simulink model "problem2b_sim_copy"  (R2024b)
settings: Solver=VariableStepAuto  StartTime=0.0  StopTime=2  FixedStep=0.04  RelTol=1e-3  AbsTol=1e-3  EnableMultiTasking=on
values from neighbouring files (symbols this model uses):
  body_a = 0.25    [Task2_up_down.m]    (also in problem2b.m; problem2b_v2.m; problem2b_v3.m; problem2b_v5.m)
  body_b = 0.15    [Task2_up_down.m]    (also in problem2b.m; problem2b_v2.m; problem2b_v3.m; problem2b_v5.m)
  body_M = 8    [Task2_up_down.m]    (also in problem2b.m; problem2b_v2.m; problem2b_v3.m; problem2b_v5.m)
  dt = 0.4    [Task2_up_down.m]    (also in problem2b.m; problem2b_v2.m = 0.05; problem2b_v3.m = 0.04; problem2b_v5.m = 0.04)
  I_body = 1/12 * body_M * (body_a^2 + body_b^2)    (= 0.0566666666667)    [Task2_up_down.m]    (also in problem2b.m; problem2b_v2.m; problem2b_v3.m; problem2b_v5.m)
  leg_l = 0.22    [Task2_up_down.m]    (also in problem2b.m; problem2b_v2.m; problem2b_v3.m; problem2b_v5.m)
  leg_m = 0.25    [Task2_up_down.m]    (also in problem2b.m; problem2b_v2.m; problem2b_v3.m; problem2b_v5.m)
  N = 5    [Task2_up_down.m]    (also in problem2b.m; problem2b_v2.m; problem2b_v3.m = 10; problem2b_v5.m = 10)
  q0 = [-pi/3; pi/2; -pi/6; pi/2]    [Task2_up_down.m]    (also in problem2b.m; problem2b_v2.m; problem2b_v3.m; problem2b_v4.m)
  x0 = 0    [Task2_up_down.m]    (also in problem2b.m; problem2b_v2.m; problem2b_v3.m; problem2b_v4.m)
  y0 = 0.45    [Task2_up_down.m]    (also in problem2b.m; problem2b_v2.m; problem2b_v3.m; problem2b_v4.m)
undefined symbols (not defined in the file or in its folder): X, Y, Z
libraries: sm_lib x17, nesl_utility x14
settings Model: Creator=zhaoshuai  LastModifiedBy=zhaoshuai
settings SolverCC: AutoScaleAbsTol=off  AlgebraicLoopSolver=TrustRegion  MaxZcPerStep=1
settings DataIOCC: LimitDataPoints=on  MaxDataPoints=10000
settings OptimizationCC: ReuseModelBlockBuffer=off  LifeSpan=inf
settings DebuggingCC: UnconnectedInputMsg=warning  UnconnectedOutputMsg=warning  UnconnectedLineMsg=warning  AllowSymbolicDim=off  SubsystemReferenceDiagnosticForUnitTest=warning  SFUnexpectedBacktrackingDiag=warning  SFNoUnconditionalDefaultTransitionDiag=warning  SFExecutionAtInitializationDiag=none  ArithmeticOperatorsInVariantConditions=warning
settings ModelReferenceCC: EnableRefExpFcnMdlSchedulingChecks=on
settings SFSimCC: SimUseLocalCustomCode=off  CustomCodeUndefinedFunction=UseInterfaceOnly
settings RTWCC: RTWUseLocalCustomCode=off  GPUComputeCapability=3.5  DLArmComputeVersion=19.05
settings CodeAppCC: StateflowObjectComments=on
settings GRTTargetCC: TargetLangStandard=C89/C90 (ANSI)
settings ConfigComp: CovMetricSettings=dw  CovSaveCumulativeToWorkspaceVar=on  CovSaveSingleToWorkspaceVar=on  CovExternalEMLEnable=off  CovSFcnEnable=off
settings SimscapeCC: SimscapeLogType=all  SimscapeLogSimulationStatistics=on  SimscapeLogDataHistory=10000

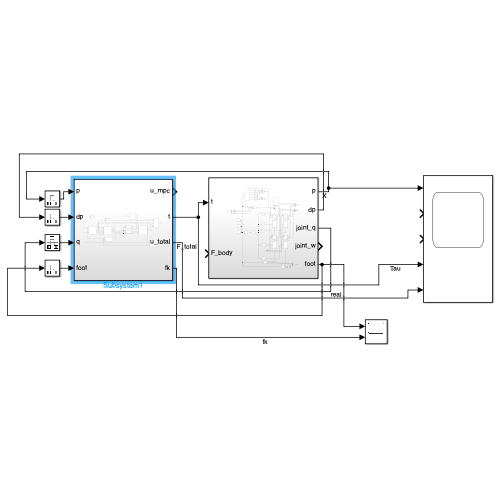
[thumbnail: Simulink's stored preview of the top-level diagram]
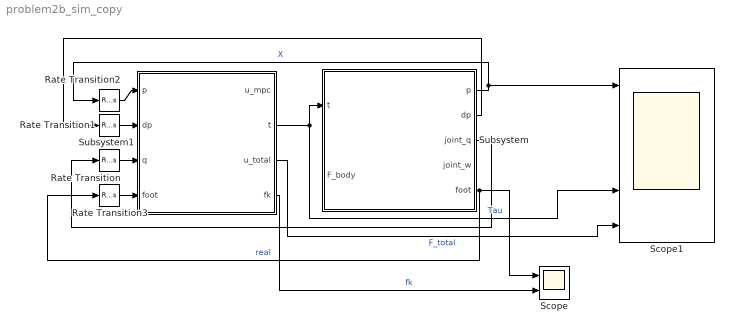
== system problem2b_sim_copy ==
  Rate Transition{,1..3} (4 alike) : RateTransition  OutPortSampleTime=dt
  Scope : Scope  NumInputPorts=2
  Scope1 : Scope  NumInputPorts=5
  Subsystem : Subsystem
  Subsystem1 : Subsystem
  wires:
  Subsystem/1(p) -> Rate Transition2/1, Scope1/1  "X"
  Subsystem1/2(t) -> Subsystem/1(t), Scope1/4  "Tau"
  Subsystem/3(joint_q) -> Rate Transition/1
  Subsystem/2(dp) -> Rate Transition1/1
  Subsystem1/3(u_total) -> Scope1/5  "F_total"
  Subsystem1/4(fk) -> Scope/2  "fk"
  Subsystem/5(foot) -> Rate Transition3/1, Scope/1  "real"
  Rate Transition/1 -> Subsystem1/3(q)
  Rate Transition1/1 -> Subsystem1/2(dp)
  Rate Transition2/1 -> Subsystem1/1(p)
  Rate Transition3/1 -> Subsystem1/4(foot)

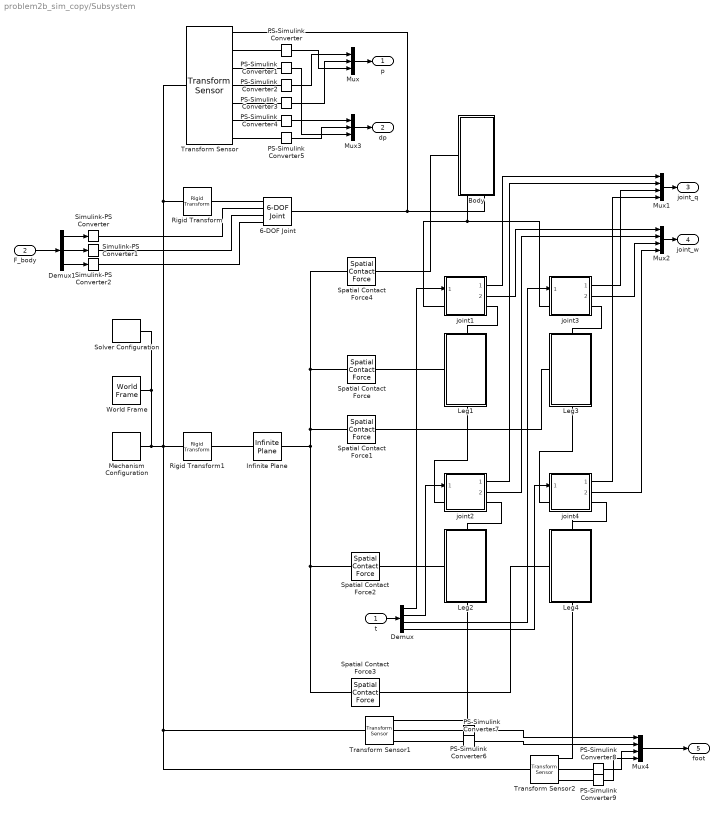
== system problem2b_sim_copy/Subsystem ==
  t : Inport
  F_body : Inport  Port=2
  6-DOF Joint : sm_lib/Joints/6-DOF Joint  JointMode=Normal  CompositeWrenchDir=FollowerOnBase  CompositeWrenchFrame=BaseFrame  SenseConstraintForce=off  SenseConstraintTorque=off  SenseTotalForce=off  SenseTotalTorque=off  PxPositionTargetSpecify=off  PxPositionTargetPriority=High  PxPositionTargetValue=0  PxPositionTargetValueUnits=m  PxVelocityTargetSpecify=off  PxVelocityTargetPriority=High  PxVelocityTargetValue=0  PxVelocityTargetValueUnits=m/s  PxEquilibriumPosition=0  PxEquilibriumPositionUnits=m  PxSpringStiffness=0  PxSpringStiffnessUnits=N/m  PxDampingCoefficient=0  PxDampingCoefficientUnits=N/(m/s)  PxLowerLimitSpecify=off  PxLowerLimitBound=-1  PxLowerLimitBoundUnits=m  PxLowerLimitStiffness=1e6  PxLowerLimitStiffnessUnits=N/m  PxLowerLimitDamping=1e3  PxLowerLimitDampingUnits=N/(m/s)  PxLowerLimitTransitionRegionWidth=1e-4  PxLowerLimitTransitionRegionWidthUnits=m  PxUpperLimitSpecify=off  PxUpperLimitBound=1  PxUpperLimitBoundUnits=m  PxUpperLimitStiffness=1e6  PxUpperLimitStiffnessUnits=N/m  PxUpperLimitDamping=1e3  PxUpperLimitDampingUnits=N/(m/s)  PxUpperLimitTransitionRegionWidth=1e-4  PxUpperLimitTransitionRegionWidthUnits=m  PxTorqueActuationMode=InputTorque  PxMotionActuationMode=ComputedMotion  PxSensePosition=off  PxSenseVelocity=off  PxSenseAcceleration=off  PxSenseTorqueForce=off  PxSenseLowerLimitTorqueForce=off  PxSenseUpperLimitTorqueForce=off  PyPositionTargetSpecify=off  PyPositionTargetPriority=High  PyPositionTargetValue=0  PyPositionTargetValueUnits=m  PyVelocityTargetSpecify=off  PyVelocityTargetPriority=High  PyVelocityTargetValue=0  PyVelocityTargetValueUnits=m/s  PyEquilibriumPosition=0  PyEquilibriumPositionUnits=m  PySpringStiffness=0  PySpringStiffnessUnits=N/m  PyDampingCoefficient=0  PyDampingCoefficientUnits=N/(m/s)  PyLowerLimitSpecify=off  PyLowerLimitBound=-1  PyLowerLimitBoundUnits=m  PyLowerLimitStiffness=1e6  PyLowerLimitStiffnessUnits=N/m  PyLowerLimitDamping=1e3  PyLowerLimitDampingUnits=N/(m/s)  PyLowerLimitTransitionRegionWidth=1e-4  PyLowerLimitTransitionRegionWidthUnits=m  PyUpperLimitSpecify=off  PyUpperLimitBound=1  PyUpperLimitBoundUnits=m  PyUpperLimitStiffness=1e6  PyUpperLimitStiffnessUnits=N/m  PyUpperLimitDamping=1e3  PyUpperLimitDampingUnits=N/(m/s)  PyUpperLimitTransitionRegionWidth=1e-4  PyUpperLimitTransitionRegionWidthUnits=m  PyTorqueActuationMode=InputTorque  PyMotionActuationMode=ComputedMotion  PySensePosition=off  PySenseVelocity=off  PySenseAcceleration=off  PySenseTorqueForce=off  PySenseLowerLimitTorqueForce=off  PySenseUpperLimitTorqueForce=off  PzPositionTargetSpecify=off  PzPositionTargetPriority=High  PzPositionTargetValue=0  PzPositionTargetValueUnits=m  PzVelocityTargetSpecify=off  PzVelocityTargetPriority=High  PzVelocityTargetValue=0  PzVelocityTargetValueUnits=m/s  PzEquilibriumPosition=0  PzEquilibriumPositionUnits=m  PzSpringStiffness=0  PzSpringStiffnessUnits=N/m  PzDampingCoefficient=0  PzDampingCoefficientUnits=N/(m/s)  PzLowerLimitSpecify=off  PzLowerLimitBound=-1  PzLowerLimitBoundUnits=m  PzLowerLimitStiffness=1e6  PzLowerLimitStiffnessUnits=N/m  PzLowerLimitDamping=1e3  PzLowerLimitDampingUnits=N/(m/s)  PzLowerLimitTransitionRegionWidth=1e-4  PzLowerLimitTransitionRegionWidthUnits=m  PzUpperLimitSpecify=off  PzUpperLimitBound=1  PzUpperLimitBoundUnits=m  PzUpperLimitStiffness=1e6  PzUpperLimitStiffnessUnits=N/m  PzUpperLimitDamping=1e3  PzUpperLimitDampingUnits=N/(m/s)  PzUpperLimitTransitionRegionWidth=1e-4  PzUpperLimitTransitionRegionWidthUnits=m  PzTorqueActuationMode=NoTorque  PzMotionActuationMode=ComputedMotion  PzSensePosition=off  PzSenseVelocity=off  PzSenseAcceleration=off  PzSenseTorqueForce=off  PzSenseLowerLimitTorqueForce=off  PzSenseUpperLimitTorqueForce=off  SphPositionTargetSpecify=off  SphPositionTargetPriority=High  SphPositionTargetRotationMethod=None  SphPositionTargetFollAlignAxisA=+X  SphPositionTargetBaseAlignAxisA=+Y  SphPositionTargetFollAlignAxisB=+Y  SphPositionTargetBaseAlignAxisB=+Z  SphPositionTargetRotationStandardAxis=+Z  SphPositionTargetRotationAngle=0.0  SphPositionTargetRotationAngleUnits=deg  SphPositionTargetRotationArbitraryAxis=[0 0 1]  SphPositionTargetRotationSequenceAxes=FollowerAxes  SphPositionTargetRotationSequence=XYX  SphPositionTargetRotationSequenceAngles=[0 0 0]  SphPositionTargetRotationSequenceAnglesUnits=deg  SphPositionTargetRotationMatrix=[1 0 0; 0 1 0; 0 0 1]  SphPositionTargetQuaternion=[1 0 0 0]  SphVelocityTargetSpecify=off  SphVelocityTargetPriority=High  SphVelocityTargetValue=[0 0 0]  SphVelocityTargetValueUnits=deg/s  SphVelocityTargetInFollowerFrame=on  SphEqPosRotationMethod=None  SphEqPosFollAlignAxisA=+X  SphEqPosBaseAlignAxisA=+Y  SphEqPosFollAlignAxisB=+Y  SphEqPosBaseAlignAxisB=+Z  SphEqPosRotationStandardAxis=+Z  SphEqPosRotationAngle=0.0  SphEqPosRotationAngleUnits=deg  SphEqPosRotationArbitraryAxis=[0 0 1]  SphEqPosRotationSequenceAxes=FollowerAxes  SphEqPosRotationSequence=XYX  SphEqPosRotationSequenceAngles=[0 0 0]  SphEqPosRotationSequenceAnglesUnits=deg  SphEqPosRotationMatrix=[1 0 0; 0 1 0; 0 0 1]  SphEqPosQuaternion=[1 0 0 0]  SphSpringStiffness=0  SphSpringStiffnessUnits=N*m/deg  SphDampingCoefficient=0  SphDampingCoefficientUnits=N*m/(deg/s)  SphLowerLimitSpecify=off  SphLowerLimitBound=15  SphLowerLimitBoundUnits=deg  SphLowerLimitStiffness=1e4  SphLowerLimitStiffnessUnits=N*m/deg  SphLowerLimitDamping=10  SphLowerLimitDampingUnits=N*m/(deg/s)  SphLowerLimitTransitionRegionWidth=0.1  SphLowerLimitTransitionRegionWidthUnits=deg  SphUpperLimitSpecify=off  SphUpperLimitBound=45  SphUpperLimitBoundUnits=deg  SphUpperLimitStiffness=1e4  SphUpperLimitStiffnessUnits=N*m/deg  SphUpperLimitDamping=10  SphUpperLimitDampingUnits=N*m/(deg/s)  SphUpperLimitTransitionRegionWidth=0.1  SphUpperLimitTransitionRegionWidthUnits=deg  SphTorqueActuationMode=InputTorque  SphActuateTorqueX=off  SphActuateTorqueY=off  SphActuateTorqueZ=on  SphActuateTorque=off  SphActuationFrame=BaseFrame  SphSensePosition=off  SphSenseVelocityX=off  SphSenseVelocityY=off  SphSenseVelocityZ=off  SphSenseVelocity=off  SphSenseAccelerationX=off  SphSenseAccelerationY=off  SphSenseAccelerationZ=off  SphSenseAcceleration=off  SphSenseLowerLimitTorqueMag=off  SphSenseUpperLimitTorqueMag=off  SphSensingFrame=BaseFrame
  Body : Subsystem  mask{a=body_a, b=body_b, m=body_M}
      settings: PortSchema="{\"entries\":[{\"content\":{\"sides\":[{\"content\":{\"connectorIds\":[\"LConn1\"]},\"type\":\"ConnectorPlacement.EquallySpacedRectSide\",\"uuid\":\"ef732868-a6ed-4fe4-817e-f9b9b43bcca9\"},{\"content\":{\"side\":\"RIGHT\"},\"type\":\"ConnectorPlacement.EquallySpacedRectSide\",\"uuid\":\"7258e0b6-9c16-4231-a684-803b12dc5dbb\"},{\"content\":{\"side\":\"TOP\"},\"type\":\"ConnectorPlacement.EquallySpacedRectSide\",\"uuid\":\"2620e2ed-2a50-4d1a-a22a-343a0fd0709a\"},{\"content\":{\"connectorIds\":[\"RConn1\",\"RConn2\"],\"side\":\"BOTTOM\"},\"type\":\"ConnectorPlacement.EquallySpacedRectSide\",\"uuid\":\"f7732c02-537d-4265-8e0b-5f0f93bf643f\"}]},\"type\":\"ConnectorPlacement.EquallySpacedConnector\",\"uuid\":\"ce80c5c0-e66c-4c1b-82fb-a63bf0c6251e\"}],\"packageUris\":[\"http://schema.mathworks.com/mf0/Connector/R2020b\"],\"version\":\"1.0\"}"
      mask DialogControl ParameterGroupVar Prompt: 参数
  Demux : Demux
  Demux1 : Demux  Outputs=3
  Infinite Plane : sm_lib/Curves and Surfaces/Infinite Plane  GraphicType=Rectangle  GraphicPlaneWidth=0.5  GraphicPlaneWidthUnits=m  GraphicPlaneHeight=0.5  GraphicPlaneHeightUnits=m  GraphicVisPropType=SimpleVisualProperties  GraphicDiffuseColor=[0.5 0.5 0.5]  GraphicOpacity=0.25  GraphicSpecularColor=[0.5 0.5 0.5 1.0]  GraphicAmbientColor=[0.15 0.15 0.15 1.0]  GraphicEmissiveColor=[0.0 0.0 0.0 1.0]  GraphicShininess=75
  Leg1 : Subsystem  ReferencedSubsystem=Leg  m=leg_m  l=leg_l  R=0.18  G=0.41  B=0.76
      settings: PortSchema="{\"entries\":[{\"content\":{\"sides\":[{\"content\":{\"connectorIds\":[\"LConn1\"]},\"type\":\"ConnectorPlacement.EquallySpacedRectSide\",\"uuid\":\"488f091b-67f3-4641-8360-22ce5240ae7f\"},{\"content\":{\"side\":\"RIGHT\"},\"type\":\"ConnectorPlacement.EquallySpacedRectSide\",\"uuid\":\"4ff6c1cd-91cf-49f0-96c7-c99ee0019842\"},{\"content\":{\"connectorIds\":[\"LConn2\"],\"side\":\"TOP\"},\"type\":\"ConnectorPlacement.EquallySpacedRectSide\",\"uuid\":\"5df597c1-c8f5-454c-942a-dba3b237f7c5\"},{\"content\":{\"connectorIds\":[\"RConn1\"],\"side\":\"BOTTOM\"},\"type\":\"ConnectorPlacement.EquallySpacedRectSide\",\"uuid\":\"edc5bfa2-1e88-4f9a-b06d-0f55ccbe67a8\"}]},\"type\":\"ConnectorPlacement.EquallySpacedConnector\",\"uuid\":\"24af63f5-949f-4fa1-b6b5-4177f1bae9a2\"}],\"packageUris\":[\"http://schema.mathworks.com/mf0/Connector/R2020b\"],\"version\":\"1.0\"}"
  Leg2 : Subsystem  ReferencedSubsystem=Leg  m=leg_m  l=leg_l  R=0.82  G=0.28  B=0
      settings: PortSchema="{\"entries\":[{\"content\":{\"sides\":[{\"content\":{\"connectorIds\":[\"LConn1\"]},\"type\":\"ConnectorPlacement.EquallySpacedRectSide\",\"uuid\":\"488f091b-67f3-4641-8360-22ce5240ae7f\"},{\"content\":{\"side\":\"RIGHT\"},\"type\":\"ConnectorPlacement.EquallySpacedRectSide\",\"uuid\":\"4ff6c1cd-91cf-49f0-96c7-c99ee0019842\"},{\"content\":{\"connectorIds\":[\"LConn2\"],\"side\":\"TOP\"},\"type\":\"ConnectorPlacement.EquallySpacedRectSide\",\"uuid\":\"5df597c1-c8f5-454c-942a-dba3b237f7c5\"},{\"content\":{\"connectorIds\":[\"RConn1\"],\"side\":\"BOTTOM\"},\"type\":\"ConnectorPlacement.EquallySpacedRectSide\",\"uuid\":\"edc5bfa2-1e88-4f9a-b06d-0f55ccbe67a8\"}]},\"type\":\"ConnectorPlacement.EquallySpacedConnector\",\"uuid\":\"24af63f5-949f-4fa1-b6b5-4177f1bae9a2\"}],\"packageUris\":[\"http://schema.mathworks.com/mf0/Connector/R2020b\"],\"version\":\"1.0\"}"
  Leg3 : Subsystem  ReferencedSubsystem=Leg  m=leg_m  l=leg_l  R=0.31  G=0.64  B=0.18
      settings: PortSchema="{\"entries\":[{\"content\":{\"sides\":[{\"content\":{\"connectorIds\":[\"LConn1\"]},\"type\":\"ConnectorPlacement.EquallySpacedRectSide\",\"uuid\":\"488f091b-67f3-4641-8360-22ce5240ae7f\"},{\"content\":{\"side\":\"RIGHT\"},\"type\":\"ConnectorPlacement.EquallySpacedRectSide\",\"uuid\":\"4ff6c1cd-91cf-49f0-96c7-c99ee0019842\"},{\"content\":{\"connectorIds\":[\"LConn2\"],\"side\":\"TOP\"},\"type\":\"ConnectorPlacement.EquallySpacedRectSide\",\"uuid\":\"5df597c1-c8f5-454c-942a-dba3b237f7c5\"},{\"content\":{\"connectorIds\":[\"RConn1\"],\"side\":\"BOTTOM\"},\"type\":\"ConnectorPlacement.EquallySpacedRectSide\",\"uuid\":\"edc5bfa2-1e88-4f9a-b06d-0f55ccbe67a8\"}]},\"type\":\"ConnectorPlacement.EquallySpacedConnector\",\"uuid\":\"24af63f5-949f-4fa1-b6b5-4177f1bae9a2\"}],\"packageUris\":[\"http://schema.mathworks.com/mf0/Connector/R2020b\"],\"version\":\"1.0\"}"
  Leg4 : Subsystem  ReferencedSubsystem=Leg  m=leg_m  l=leg_l  R=1  G=0.84  B=0.27
      settings: PortSchema="{\"entries\":[{\"content\":{\"sides\":[{\"content\":{\"connectorIds\":[\"LConn1\"]},\"type\":\"ConnectorPlacement.EquallySpacedRectSide\",\"uuid\":\"488f091b-67f3-4641-8360-22ce5240ae7f\"},{\"content\":{\"side\":\"RIGHT\"},\"type\":\"ConnectorPlacement.EquallySpacedRectSide\",\"uuid\":\"4ff6c1cd-91cf-49f0-96c7-c99ee0019842\"},{\"content\":{\"connectorIds\":[\"LConn2\"],\"side\":\"TOP\"},\"type\":\"ConnectorPlacement.EquallySpacedRectSide\",\"uuid\":\"5df597c1-c8f5-454c-942a-dba3b237f7c5\"},{\"content\":{\"connectorIds\":[\"RConn1\"],\"side\":\"BOTTOM\"},\"type\":\"ConnectorPlacement.EquallySpacedRectSide\",\"uuid\":\"edc5bfa2-1e88-4f9a-b06d-0f55ccbe67a8\"}]},\"type\":\"ConnectorPlacement.EquallySpacedConnector\",\"uuid\":\"24af63f5-949f-4fa1-b6b5-4177f1bae9a2\"}],\"packageUris\":[\"http://schema.mathworks.com/mf0/Connector/R2020b\"],\"version\":\"1.0\"}"
  Mechanism Configuration : sm_lib/Utilities/Mechanism Configuration  UniformGravity=Constant  GravityVector=[0 -9.80665 0]  GravityVectorUnits=m/s^2  LinearizationDelta=0.001  JointModeTransitionNonlinearIterations=2
  Mux : Mux  Inputs=3
  Mux1 : Mux
  Mux2 : Mux
  Mux3 : Mux  Inputs=3
  Mux4 : Mux
  PS-Simulink Converter{,1..9} (10 alike) : nesl_utility/PS-Simulink Converter  PhysicalDomain=network_engine_domain  SubClassName=ps_output  LeftPortType=input  RightPortType=output  PseudoPeriodic=off  Frequencies=[]  VectorFormat=inherit  Unit=inherit  AffineConversion=off
  Rigid Transform : sm_lib/Frames and Transforms/Rigid Transform  RotationMethod=None  FollAlignAxisA=+X  BaseAlignAxisA=+Y  FollAlignAxisB=+Y  BaseAlignAxisB=+Z  RotationStandardAxis=+Z  RotationAngle=0.0  RotationAngleUnits=deg  RotationArbitraryAxis=[0 0 1]  RotationSequenceAxes=FollowerAxes  RotationSequence=XYX  RotationSequenceAngles=[0 0 0]  RotationSequenceAnglesUnits=deg  RotationMatrix=[1 0 0; 0 1 0; 0 0 1]  Quaternion=[1 0 0 0]  TranslationMethod=Cartesian  TranslationCartesianOffset=[x0 y0 0]  TranslationCartesianOffsetUnits=m  TranslationStandardAxis=+Y  TranslationStandardOffset=y0  TranslationStandardOffsetUnits=m  TranslationROffset=0  TranslationROffsetUnits=m  TranslationThetaOffset=0  TranslationThetaOffsetUnits=deg  TranslationZOffset=0  TranslationZOffsetUnits=m
  Rigid Transform1 : sm_lib/Frames and Transforms/Rigid Transform  RotationMethod=AlignedAxes  FollAlignAxisA=+X  BaseAlignAxisA=+Z  FollAlignAxisB=+Y  BaseAlignAxisB=+X  RotationStandardAxis=+Z  RotationAngle=0.0  RotationAngleUnits=deg  RotationArbitraryAxis=[0 0 1]  RotationSequenceAxes=FollowerAxes  RotationSequence=XYX  RotationSequenceAngles=[0 0 0]  RotationSequenceAnglesUnits=deg  RotationMatrix=[1 0 0; 0 1 0; 0 0 1]  Quaternion=[1 0 0 0]  TranslationMethod=None  TranslationCartesianOffset=[0 0 0]  TranslationCartesianOffsetUnits=m  TranslationStandardAxis=+Z  TranslationStandardOffset=0  TranslationStandardOffsetUnits=m  TranslationROffset=0  TranslationROffsetUnits=m  TranslationThetaOffset=0  TranslationThetaOffsetUnits=deg  TranslationZOffset=0  TranslationZOffsetUnits=m
  Simulink-PS Converter : nesl_utility/Simulink-PS Converter  PhysicalDomain=network_engine_domain  SubClassName=ps_input  LeftPortType=input  RightPortType=output  PseudoPeriodic=off  Frequencies=[]  NoiseDistribution=none  NoiseParameters=[]  Unit=1  AffineConversion=off  FilteringAndDerivatives=provide  SimscapeFilterOrder=1  InputFilterTimeConstant=0.001  UdotUserProvided=0
  Simulink-PS Converter1 : nesl_utility/Simulink-PS Converter  PhysicalDomain=network_engine_domain  SubClassName=ps_input  LeftPortType=input  RightPortType=output  PseudoPeriodic=off  Frequencies=[]  NoiseDistribution=none  NoiseParameters=[]  Unit=1  AffineConversion=off  FilteringAndDerivatives=provide  SimscapeFilterOrder=1  InputFilterTimeConstant=0.001  UdotUserProvided=0
  Simulink-PS Converter2 : nesl_utility/Simulink-PS Converter  PhysicalDomain=network_engine_domain  SubClassName=ps_input  LeftPortType=input  RightPortType=output  PseudoPeriodic=off  Frequencies=[]  NoiseDistribution=none  NoiseParameters=[]  Unit=1  AffineConversion=off  FilteringAndDerivatives=provide  SimscapeFilterOrder=1  InputFilterTimeConstant=0.001  UdotUserProvided=0
  Solver Configuration : nesl_utility/Solver Configuration  PhysicalDomain=network_engine_domain  SubClassName=solver  LeftPortType=input  RightPortType=generic  Tones=[]  Harmonics=[]  SimulateNoise=off  Profile=off  UseLocalSampling=off  EnableSwitchedLinearOptims=on  FrequencyDomain=off  UseCCode=off  RelTol=0.001  AbsTol=1e-06  MinStep=1e-09  ToWorkspace=off  RevertToSquareIcSolve=off  NumHomotopyIterations=100  PhasorMode=off  PhasorModeNumHarmonics=1  ConsistencySolver=NEWTON_XTOL_AFTER_FTOL  IndexReductionMethod=DerivativeReplacement  DoDC=off  ResidualTolerance=1e-09  ConsistencyTolSource=GLOBAL  ConsistencyAbsTol=0.001  ConsistencyRelTol=0.001  ConsistencyTolFactor=0.001  UseLocalSolver=off  LocalSolverChoice=NE_BACKWARD_EULER_ADVANCER  ResolveIndetEquations=on  FunctionEvalNumThread=1  LocalSolverSampleTime=0.001  DoFixedCost=off  MaxNonlinIter=3  MaxModeIter=2  ComputeImpulses=off  ImpulseIterations=2  LinearAlgebra=Sparse  LinearAlgebraNumThread=0  EquationFormulation=NE_TIME_EF  DelaysMemoryBudget=1024  AutomaticFiltering=on  FilteringTimeConstant=0.001  PartitionStorageMethod=AS_NEEDED  PartitionMemoryBudget=1024  PartitionMethod=FAST  MultibodyUseLocalSolver=off  MultibodyLocalSolverChoice=ODE1  MultibodyLocalSolverSampleTime=0.001
  Spatial Contact Force{,1..4} (5 alike) : sm_lib/Forces and Torques/Spatial Contact Force  NormalForceType=SmoothSpringDamper  NormalStiffness=1e5  NormalStiffnessUnits=N/m  NormalDamping=1e3  NormalDampingUnits=N/(m/s)  NormalTransitionRegionWidth=1e-4  NormalTransitionRegionWidthUnits=m  FrictionType=SmoothStickSlip  CoefficientOfStaticFriction=0.7  CoefficientOfDynamicFriction=0.5  FrictionalCriticalVelocity=1e-3  FrictionalCriticalVelocityUnits=m/s  SenseContactSignal=off  SensePenetrationDepth=off  SenseSeparationDistance=off  SenseNormalForceMagnitude=off  SenseFrictionalForceMagnitude=off  SenseNormalVelocity=off  SenseTangentialVelocity=off  SenseContactBaseRotation=off  SenseContactBaseTranslation=off  SenseContactFollowerRotation=off  SenseContactFollowerTranslation=off  ZeroCrossDetectContactStartAndEnd=off
  Transform Sensor : sm_lib/Frames and Transforms/Transform Sensor  MeasurementFrame=World  RotationSequence=XYX  SenseAngle=on  SenseAxis=off  SenseQ=off  SenseR=off  SenseRotationSequence=off  SenseOmegaX=off  SenseOmegaY=off  SenseOmegaZ=on  SenseOmega=off  SenseQDot=off  SenseRDot=off  SenseRotationSequenceDot=off  SenseAlphaX=off  SenseAlphaY=off  SenseAlphaZ=off  SenseAlpha=off  SenseQDDot=off  SenseRDDot=off  SenseX=on  SenseY=on  SenseZ=off  SenseXYZ=off  SenseRad=off  SenseAzim=off  SenseDist=off  SenseInc=off  SenseXDot=on  SenseYDot=on  SenseZDot=off  SenseXYZDot=off  SenseRadDot=off  SenseAzimDot=off  SenseDistDot=off  SenseIncDot=off  SenseXDDot=off  SenseYDDot=off  SenseZDDot=off  SenseXYZDDot=off  SenseRadDDot=off  SenseAzimDDot=off  SenseDistDDot=off  SenseIncDDot=off
  Transform Sensor1 : sm_lib/Frames and Transforms/Transform Sensor  MeasurementFrame=World  RotationSequence=XYX  SenseAngle=off  SenseAxis=off  SenseQ=off  SenseR=off  SenseRotationSequence=off  SenseOmegaX=off  SenseOmegaY=off  SenseOmegaZ=off  SenseOmega=off  SenseQDot=off  SenseRDot=off  SenseRotationSequenceDot=off  SenseAlphaX=off  SenseAlphaY=off  SenseAlphaZ=off  SenseAlpha=off  SenseQDDot=off  SenseRDDot=off  SenseX=on  SenseY=on  SenseZ=off  SenseXYZ=off  SenseRad=off  SenseAzim=off  SenseDist=off  SenseInc=off  SenseXDot=off  SenseYDot=off  SenseZDot=off  SenseXYZDot=off  SenseRadDot=off  SenseAzimDot=off  SenseDistDot=off  SenseIncDot=off  SenseXDDot=off  SenseYDDot=off  SenseZDDot=off  SenseXYZDDot=off  SenseRadDDot=off  SenseAzimDDot=off  SenseDistDDot=off  SenseIncDDot=off
  Transform Sensor2 : sm_lib/Frames and Transforms/Transform Sensor  MeasurementFrame=World  RotationSequence=XYX  SenseAngle=off  SenseAxis=off  SenseQ=off  SenseR=off  SenseRotationSequence=off  SenseOmegaX=off  SenseOmegaY=off  SenseOmegaZ=off  SenseOmega=off  SenseQDot=off  SenseRDot=off  SenseRotationSequenceDot=off  SenseAlphaX=off  SenseAlphaY=off  SenseAlphaZ=off  SenseAlpha=off  SenseQDDot=off  SenseRDDot=off  SenseX=on  SenseY=on  SenseZ=off  SenseXYZ=off  SenseRad=off  SenseAzim=off  SenseDist=off  SenseInc=off  SenseXDot=off  SenseYDot=off  SenseZDot=off  SenseXYZDot=off  SenseRadDot=off  SenseAzimDot=off  SenseDistDot=off  SenseIncDot=off  SenseXDDot=off  SenseYDDot=off  SenseZDDot=off  SenseXYZDDot=off  SenseRadDDot=off  SenseAzimDDot=off  SenseDistDDot=off  SenseIncDDot=off
  World Frame : sm_lib/Frames and Transforms/World Frame
  joint1 : Subsystem  ReferencedSubsystem=hip  q0=q0(1)
  joint2 : Subsystem  ReferencedSubsystem=knee  q0=q0(2)
  joint3 : Subsystem  ReferencedSubsystem=hip  q0=q0(3)
  joint4 : Subsystem  ReferencedSubsystem=knee  q0=q0(4)
  p : Outport
  dp : Outport  Port=2
  joint_q : Outport  Port=3
  joint_w : Outport  Port=4
  foot : Outport  Port=5
  wires:
  Demux/4 -> joint4/1
  joint4/2 -> Mux2/4
  joint1/2 -> Mux2/1
  joint2/1 -> Mux1/2
  PS-Simulink Converter2/1 -> Mux/1
  Demux/3 -> joint3/1
  joint3/1 -> Mux1/3
  Demux/2 -> joint2/1
  t/1 -> Demux/1
  joint2/2 -> Mux2/2
  Demux/1 -> joint1/1
  joint1/1 -> Mux1/1
  joint3/2 -> Mux2/3
  Mux1/1 -> joint_q/1
  PS-Simulink Converter/1 -> Mux/3
  joint4/1 -> Mux1/4
  Mux2/1 -> joint_w/1
  PS-Simulink Converter3/1 -> Mux/2
  PS-Simulink Converter4/1 -> Mux3/1
  PS-Simulink Converter5/1 -> Mux3/2
  Mux/1 -> p/1
  Mux3/1 -> dp/1
  PS-Simulink Converter1/1 -> Mux3/3
  F_body/1 -> Demux1/1
  Demux1/1 -> Simulink-PS Converter/1
  Demux1/2 -> Simulink-PS Converter1/1
  Demux1/3 -> Simulink-PS Converter2/1
  PS-Simulink Converter6/1 -> Mux4/1
  PS-Simulink Converter7/1 -> Mux4/2
  PS-Simulink Converter8/1 -> Mux4/3
  PS-Simulink Converter9/1 -> Mux4/4
  Mux4/1 -> foot/1
  connections:
  Spatial Contact Force1/RConn1 -- Leg3/LConn1
  Transform Sensor/RConn1 -- Body/RConn2 -- 6-DOF Joint/RConn1
  joint2/RConn1 -- Leg2/LConn2
  joint3/RConn1 -- Leg3/LConn2
  joint2/LConn1 -- Leg1/RConn1
  PS-Simulink Converter/LConn1 -- Transform Sensor/RConn2
  PS-Simulink Converter2/LConn1 -- Transform Sensor/RConn4
  joint1/RConn1 -- Leg1/LConn2
  Rigid Transform/RConn1 -- 6-DOF Joint/LConn1
  Infinite Plane/RConn1 -- Spatial Contact Force3/LConn1 -- Spatial Contact Force2/LConn1 -- Spatial Contact Force1/LConn1 -- Spatial Contact Force/LConn1 -- Spatial Contact Force4/LConn1
  Body/LConn1 -- Spatial Contact Force4/RConn1
  Spatial Contact Force/RConn1 -- Leg1/LConn1
  Body/RConn1 -- joint1/LConn1 -- joint3/LConn1
  PS-Simulink Converter1/LConn1 -- Transform Sensor/RConn3
  Infinite Plane/LConn1 -- Rigid Transform1/RConn1
  Leg4/LConn2 -- joint4/RConn1
  joint4/LConn1 -- Leg3/RConn1
  Mechanism Configuration/RConn1 -- Transform Sensor2/LConn1 -- Transform Sensor1/LConn1 -- Transform Sensor/LConn1 -- Rigid Transform/LConn1 -- Rigid Transform1/LConn1 -- World Frame/RConn1 -- Solver Configuration/RConn1
  PS-Simulink Converter3/LConn1 -- Transform Sensor/RConn5
  PS-Simulink Converter4/LConn1 -- Transform Sensor/RConn6
  Transform Sensor/RConn7 -- PS-Simulink Converter5/LConn1
  Simulink-PS Converter/RConn1 -- 6-DOF Joint/LConn2
  6-DOF Joint/LConn3 -- Simulink-PS Converter1/RConn1
  Simulink-PS Converter2/RConn1 -- 6-DOF Joint/LConn4
  Leg4/LConn1 -- Spatial Contact Force3/RConn1
  Leg2/LConn1 -- Spatial Contact Force2/RConn1
  Transform Sensor1/RConn1 -- Leg2/RConn1
  Transform Sensor2/RConn1 -- Leg4/RConn1
  Transform Sensor1/RConn2 -- PS-Simulink Converter6/LConn1
  Transform Sensor1/RConn3 -- PS-Simulink Converter7/LConn1
  PS-Simulink Converter8/LConn1 -- Transform Sensor2/RConn2
  PS-Simulink Converter9/LConn1 -- Transform Sensor2/RConn3

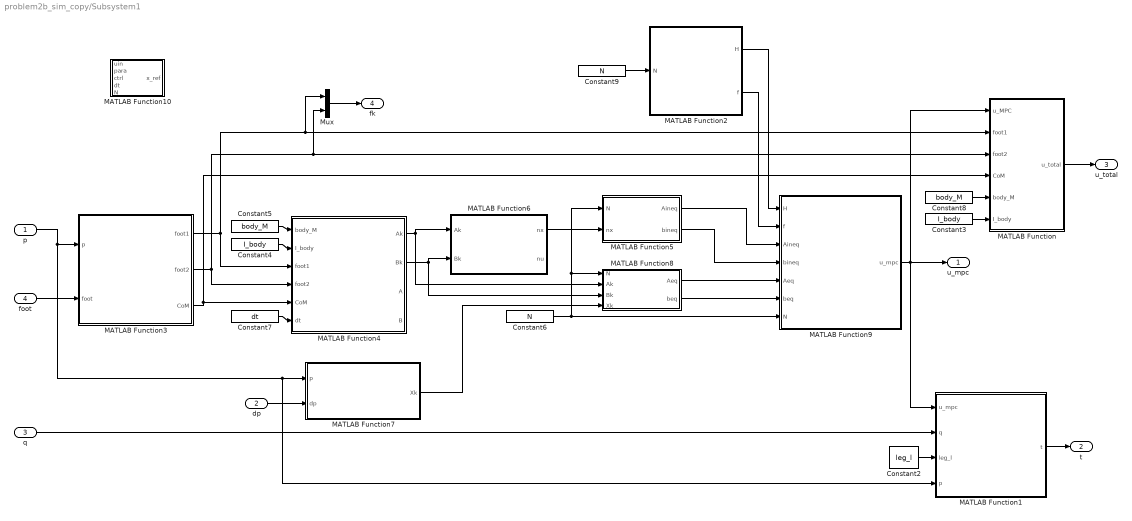
== system problem2b_sim_copy/Subsystem1 ==
  p : Inport
  dp : Inport  Port=2
  q : Inport  Port=3
  foot : Inport  Port=4
  Constant2 : Constant  Value=leg_l
  Constant3 : Constant  Value=I_body
  Constant4 : Constant  Value=I_body
  Constant5 : Constant  Value=body_M
  Constant6 : Constant  Value=N
  Constant7 : Constant  Value=dt
  Constant8 : Constant  Value=body_M
  Constant9 : Constant  Value=N
  MATLAB Function : MATLAB Function  TreatAsAtomicUnit=on
  MATLAB Function1 : MATLAB Function  TreatAsAtomicUnit=on
  MATLAB Function10 : MATLAB Function  TreatAsAtomicUnit=on
  MATLAB Function2 : MATLAB Function  TreatAsAtomicUnit=on
  MATLAB Function3 : MATLAB Function  TreatAsAtomicUnit=on
  MATLAB Function4 : MATLAB Function  TreatAsAtomicUnit=on
  MATLAB Function5 : MATLAB Function  TreatAsAtomicUnit=on
  MATLAB Function6 : MATLAB Function  TreatAsAtomicUnit=on
  MATLAB Function7 : MATLAB Function  TreatAsAtomicUnit=on
  MATLAB Function8 : MATLAB Function  TreatAsAtomicUnit=on
  MATLAB Function9 : MATLAB Function  TreatAsAtomicUnit=on
  Mux : Mux  Inputs=2
  u_mpc : Outport
  t : Outport  Port=2
  u_total : Outport  Port=3
  fk : Outport  Port=4
  wires:
  dp/1 -> MATLAB Function7/2(dp)
  MATLAB Function1/1(t) -> t/1
  MATLAB Function3/2(foot2) -> MATLAB Function/3(foot2), Mux/2, MATLAB Function4/4(foot2)
  q/1 -> MATLAB Function1/2(q)
  MATLAB Function3/3(CoM) -> MATLAB Function/4(CoM), MATLAB Function4/5(CoM)
  p/1 -> MATLAB Function1/4(p), MATLAB Function7/1(p), MATLAB Function3/1(p)
  Constant2/1 -> MATLAB Function1/3(leg_l)
  Constant4/1 -> MATLAB Function4/2(I_body)
  MATLAB Function3/1(foot1) -> MATLAB Function4/3(foot1), MATLAB Function/2(foot1), Mux/1
  Constant7/1 -> MATLAB Function4/6(dt)
  MATLAB Function7/1(Xk) -> MATLAB Function8/4(Xk)
  MATLAB Function9/1(u_mpc) -> MATLAB Function1/1(u_mpc), u_mpc/1, MATLAB Function/1(u_MPC)
  MATLAB Function/1(u_total) -> u_total/1
  Constant8/1 -> MATLAB Function/5(body_M)
  Mux/1 -> fk/1
  Constant5/1 -> MATLAB Function4/1(body_M)
  Constant6/1 -> MATLAB Function5/1(N), MATLAB Function8/1(N), MATLAB Function9/7(N)
  Constant3/1 -> MATLAB Function/6(I_body)
  Constant9/1 -> MATLAB Function2/1(N)
  MATLAB Function2/1(H) -> MATLAB Function9/1(H)
  MATLAB Function2/2(f) -> MATLAB Function9/2(f)
  MATLAB Function4/1(Ak) -> MATLAB Function6/1(Ak), MATLAB Function8/2(Ak)
  MATLAB Function4/2(Bk) -> MATLAB Function6/2(Bk), MATLAB Function8/3(Bk)
  MATLAB Function6/1(nx) -> MATLAB Function5/2(nx)
  MATLAB Function5/1(Aineq) -> MATLAB Function9/3(Aineq)
  MATLAB Function5/2(bineq) -> MATLAB Function9/4(bineq)
  MATLAB Function8/1(Aeq) -> MATLAB Function9/5(Aeq)
  MATLAB Function8/2(beq) -> MATLAB Function9/6(beq)
  foot/1 -> MATLAB Function3/2(foot)

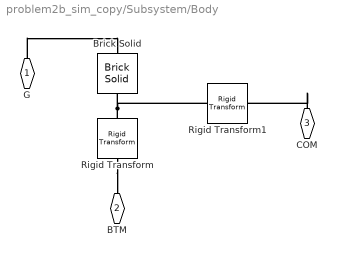
== system problem2b_sim_copy/Subsystem/Body ==
  Brick Solid : sm_lib/Body Elements/Brick Solid  BrickDimensions=[b a 0.1]  BrickDimensionsUnits=m  ExportEntireGeometry=on  InertiaType=Custom  BasedOnType=Mass  Density=1000  DensityUnits=kg/m^3  Mass=m  MassUnits=kg  CenterOfMass=[0 0 0]  CenterOfMassUnits=m  MomentsOfInertia=[1 1 1/12*m*(a^2+b^2)]  MomentsOfInertiaUnits=kg*m^2  ProductsOfInertia=[0 0 0]  ProductsOfInertiaUnits=kg*m^2  GraphicType=FromGeometry  MarkerShape=Sphere  MarkerSize=10  GraphicVisPropType=SimpleVisualProperties  GraphicDiffuseColor=[0.4 0.4 0.4]  GraphicOpacity=1.0  GraphicSpecularColor=[0.5 0.5 0.5 1.0]  GraphicAmbientColor=[0.15 0.15 0.15 1.0]  GraphicEmissiveColor=[0.0 0.0 0.0 1.0]  GraphicShininess=75  DoExposeReferenceFrame=on  SerializedFrames=<Frames/>
  Rigid Transform : sm_lib/Frames and Transforms/Rigid Transform  RotationMethod=None  FollAlignAxisA=+X  BaseAlignAxisA=+Y  FollAlignAxisB=+Y  BaseAlignAxisB=+Z  RotationStandardAxis=+Z  RotationAngle=0.0  RotationAngleUnits=deg  RotationArbitraryAxis=[0 0 1]  RotationSequenceAxes=FollowerAxes  RotationSequence=XYX  RotationSequenceAngles=[0 0 0]  RotationSequenceAnglesUnits=deg  RotationMatrix=[1 0 0; 0 1 0; 0 0 1]  Quaternion=[1 0 0 0]  TranslationMethod=StandardAxis  TranslationCartesianOffset=[0 0 0]  TranslationCartesianOffsetUnits=m  TranslationStandardAxis=-Y  TranslationStandardOffset=0.125  TranslationStandardOffsetUnits=m  TranslationROffset=0  TranslationROffsetUnits=m  TranslationThetaOffset=0  TranslationThetaOffsetUnits=deg  TranslationZOffset=0  TranslationZOffsetUnits=m
  Rigid Transform1 : sm_lib/Frames and Transforms/Rigid Transform  RotationMethod=None  FollAlignAxisA=+X  BaseAlignAxisA=+Y  FollAlignAxisB=+Y  BaseAlignAxisB=+Z  RotationStandardAxis=+Z  RotationAngle=0.0  RotationAngleUnits=deg  RotationArbitraryAxis=[0 0 1]  RotationSequenceAxes=FollowerAxes  RotationSequence=XYX  RotationSequenceAngles=[0 0 0]  RotationSequenceAnglesUnits=deg  RotationMatrix=[1 0 0; 0 1 0; 0 0 1]  Quaternion=[1 0 0 0]  TranslationMethod=None  TranslationCartesianOffset=[0 0 0]  TranslationCartesianOffsetUnits=m  TranslationStandardAxis=+Z  TranslationStandardOffset=0  TranslationStandardOffsetUnits=m  TranslationROffset=0  TranslationROffsetUnits=m  TranslationThetaOffset=0  TranslationThetaOffsetUnits=deg  TranslationZOffset=0  TranslationZOffsetUnits=m
  G : PMIOPort  Side=Left
  BTM : PMIOPort  Port=2  Side=Right
  COM : PMIOPort  Port=3  Side=Right
  connections:
  Rigid Transform/RConn1 -- BTM/RConn1
  Brick Solid/RConn1 -- Rigid Transform/LConn1 -- Rigid Transform1/LConn1
  G/RConn1 -- Brick Solid/LConn1
  COM/RConn1 -- Rigid Transform1/RConn1

== matlab function problem2b_sim_copy/Subsystem1/MATLAB Function7 ==
  data: p input; dp input; Xk output
function Xk = get_Xk(p, dp)

g = 9.81;

x = p(1); 
y = p(2); 
theta = p(3); 

vx = dp(1);
vy = dp(2); 
omega = dp(3);

Xk = [x; y; theta; vx; vy; omega; g];

end

== matlab function problem2b_sim_copy/Subsystem1/MATLAB Function9 ==
  data: H input; f input; Aineq input; bineq input; Aeq input; beq input; N input; u_mpc output
function u_mpc = MPC(H ,f, Aineq, bineq, Aeq, beq, N)

% paramters
nx = 7; 
nu = 4; 

% X0
X0 = zeros((nx + nu) * N, 1); 

% quadprog
options = optimoptions('quadprog', 'Algorithm', 'active-set', 'Display', 'none');
X_star = quadprog(H, f, Aineq, bineq, Aeq, beq, [], [], X0, options);

% 提取结果
U_pred = X_star(N*nx+1:end);   % 预测的未来 N 步输入
u_mpc = U_pred(1:nu);             % 当前优化的第一个输入

end

== matlab function problem2b_sim_copy/Subsystem1/MATLAB Function8 ==
  data: N input; Aeq output; Ak input; Bk input; Xk input; beq output
function [Aeq, beq] = eq(N, Ak, Bk, Xk)

    nx = size(Ak,1);
    
    % Define equality constraints
    Aeq_state = kron(eye(N), eye(nx)) + kron(diag(ones(N-1, 1), -1), -Ak);
    Aeq_input = kron(eye(N), -Bk);
    Aeq = [Aeq_state, Aeq_input];
    beq = [Ak * Xk; zeros(nx * (N - 1), 1)];

end

== matlab function problem2b_sim_copy/Subsystem1/MATLAB Function10 ==
  data: uin input; x_ref output; para input; ctrl input; dt input; N input
function x_ref = getReferenceTrajectory(uin, para, ctrl, dt, N)
    % Generate our target trajectory for use in MPC

    xd = [0; 0.5; 0; 0; 0; 0];
    x_ref = repmat([xd;1], 1, N);

    for i = 1:3
        for k = 2:N
            if ctrl.x_cmd(i+3) ~= 0
                x_ref(i,k) = uin(i)+ctrl.x_cmd(i+3)*((k-1)*dt);
            else
                x_ref(i,k) = ctrl.x_cmd(i);
            end
        end
    end
end

== matlab function problem2b_sim_copy/Subsystem1/MATLAB Function1 ==
  data: u_mpc input; q input; t output; leg_l input; p input
function t = ifk(u_mpc, q, leg_l, p)
    
    % 提取关节角度
    q1 = q(1);
    q2 = q(2);
    q3 = q(3);
    q4 = q(4);
    theta = p(3);

    % 创建 world frame 到 body frame 的旋转矩阵
    R_world_to_body = [cos(theta), sin(theta);
                      -sin(theta), cos(theta)];

    % 将支撑力 u_qp 转换到 body frame
    u_body = zeros(size(u_mpc));
    u_body(1:2) = R_world_to_body * u_mpc(1:2);  % 第一个腿的支撑力
    u_body(3:4) = R_world_to_body * u_mpc(3:4);  % 第二个腿的支撑力

    % 计算雅可比矩阵
    J = [leg_l*cos(q1 + q2) + leg_l*cos(q1), leg_l*cos(q1 + q2),                                  0,                  0;
         leg_l*sin(q1 + q2) + leg_l*sin(q1), leg_l*sin(q1 + q2),                                  0,                  0;
                                          0,                  0, leg_l*cos(q3 + q4) + leg_l*cos(q3), leg_l*cos(q3 + q4);
                                          0,                  0, leg_l*sin(q3 + q4) + leg_l*sin(q3), leg_l*sin(q3 + q4)];

    % 计算关节力矩 t
    t = - J' * u_body;  % 支撑力到关节力矩的转换
end

== matlab function problem2b_sim_copy/Subsystem1/MATLAB Function ==
  data: u_MPC input; u_total output; foot1 input; foot2 input; CoM input; body_M input; I_body input
function u_total = totalforce(u_MPC, foot1, foot2, CoM, body_M, I_body)
f1x = u_MPC(1);
f1y = u_MPC(2);
f2x = u_MPC(3);
f2y = u_MPC(4);

% 提取位置参数
x1 = foot1(1); y1 = foot1(2);
x2 = foot2(1); y2 = foot2(2);
xc = CoM(1); yc = CoM(2);

fx_total = f1x+f2x;
fy_total = f1y+f2y;
t_total = -f1x*(y1-yc)+f1y*(x1-xc)-f2x*(y2-yc)+f2y*(x2-xc);

u_total = [fx_total;fy_total;t_total];
end

== matlab function problem2b_sim_copy/Subsystem1/MATLAB Function2 ==
  data: H output; N input; f output
function [H, f] = cost_function(N)
    
    % Q & R
    Q = diag([200 200 800 10 10 30 1]); 
    R = diag([0.0001 0.0001 0.0001 0.0001]);    
   
    H = blkdiag(kron(eye(N), Q), kron(eye(N), R)); 

    ref = [0; 0.5; 0; 0; 0; 0; 9.81];
    f_state = repmat(-2 * Q * ref, N, 1);
    f_input = repmat([0; 0; 0; 0], N, 1); 
    f = [f_state; f_input]; 
end

== matlab function problem2b_sim_copy/Subsystem1/MATLAB Function3 ==
  data: p input; foot1 output; foot input; foot2 output; CoM output
function [foot1, foot2, CoM] = fk(p, foot)
    
    x = p(1);
    y = p(2);
    theta = p(3);

    foot1 = foot(1);
    foot2 = foot(1);
    CoM = [x, y];
end

== matlab function problem2b_sim_copy/Subsystem1/MATLAB Function4 ==
  data: body_M input; I_body input; foot1 input; foot2 input; Ak output; CoM input; Bk output; dt input; A output; B output
function [Ak, Bk, A, B] = dynamics(body_M, I_body, foot1, foot2, CoM, dt)

x1 = foot1(1); y1 = foot1(2);
x2 = foot2(1); y2 = foot2(2);
xc = CoM(1); yc = CoM(2);

g = 9.81; 

I_world = I_body; % only for 2D 

% Act
A = zeros(7,7);
A(1,4) = 1; 
A(2,5) = 1;
A(3,6) = 1; 
A(5,7) = -1; 

% Bct
B = zeros(7,4);
B(4,1) = 1 / body_M; % Fx1 
B(4,3) = 1 / body_M; % Fx2 
B(5,2) = 1 / body_M; % Fy1 
B(5,4) = 1 / body_M; % Fy2 
B(6,1) = -(y1 - yc) / I_world; % Fx1 M
B(6,2) = (x1 - xc) / I_world; % Fy1 M
B(6,3) = -(y2 - yc) / I_world; % Fx2 M
B(6,4) = (x2 - xc) / I_world; % Fy2 M

% Ak Bk
Ak = eye(size(A)) + A .* dt;
Bk = B .* dt;

end

== matlab function problem2b_sim_copy/Subsystem1/MATLAB Function5 ==
  data: N input; Aineq output; nx input; bineq output
function [Aineq, bineq] = ineq(N, nx)

    mu = 0.7;
    
    Aineq_state = zeros(nx, nx); 
    bineq_state = zeros(nx, 1);  
    
    Aineq_input = [
        0,  1,  0,  0;   % F1y ≤ 250
        0, -1,  0,  0;   % -F1y ≤ -10
        0,  0,  0,  1;   % F2y ≤ 250
        0,  0,  0, -1;   % -F2y ≤ -10
        1, -mu, 0,  0;   % F1x ≤ μ * F1y
       -1, -mu, 0,  0;   % F1x ≥ -μ * F1y
        0,  0,  1, -mu;  % F2x ≤ μ * F2y
        0,  0, -1, -mu   % F2x ≥ -μ * F2y
    ];
    bineq_input = [250; -10; 250; -10; 0; 0; 0; 0];

    % Combine constraints
    Aineq = blkdiag(kron(eye(N),Aineq_state),kron(eye(N),Aineq_input));
    bineq = [repmat(bineq_state,N,1); repmat(bineq_input,N,1)];

end

== matlab function problem2b_sim_copy/Subsystem1/MATLAB Function6 ==
  data: Ak input; nx output; Bk input; nu output
function [nx, nu] = get_dimention(Ak, Bk)

    nx = size(Ak,1);
    nu = size(Bk,2);

end
